simulink model "s_lqr_solar_tracking"  (R2017a)
settings: Solver=VariableStepAuto  StartTime=0.0  StopTime=10  RelTol=1e-3
values from neighbouring files (symbols this model uses):
  A = [(-R/L) (-k2/L) 0; (k1/J) 0 0; 0 1 0]    [lqr_solar_tracking.m]
  B = [(1/L); 0; 0]    [lqr_solar_tracking.m]
  C = [0 0 1]    [lqr_solar_tracking.m]
  K = lqr(A,B,Q,R)    [lqr_solar_tracking.m]
settings Model: Creator=NEGATIVE  LastModifiedBy=NEGATIVE

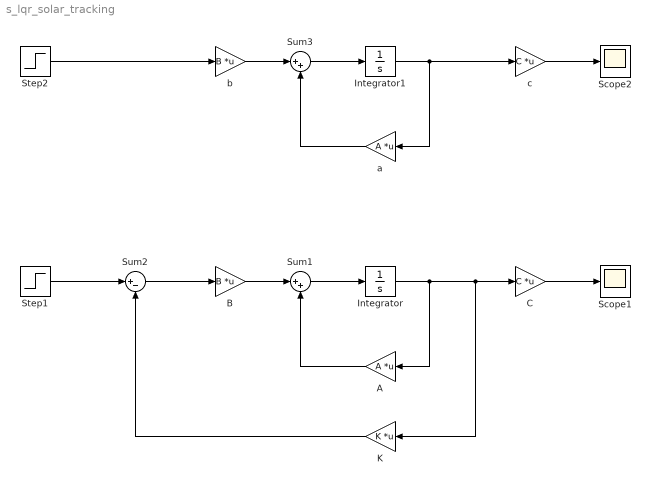
== system s_lqr_solar_tracking ==
  A : Gain  Gain=A  Multiplication=Matrix(K*u)
  B : Gain  Gain=B  Multiplication=Matrix(K*u)
  C : Gain  Gain=C  Multiplication=Matrix(K*u)
  Integrator : Integrator
  Integrator1 : Integrator
  K : Gain  Gain=K  Multiplication=Matrix(K*u)
  Scope1 : Scope
  Scope2 : Scope
  Step1 : Step  Time=0  After=24  SampleTime=0
  Step2 : Step  Time=0  After=24  SampleTime=0
  Sum1 : Sum  Inputs=|++
  Sum2 : Sum  Inputs=|+-
  Sum3 : Sum  Inputs=|++
  a : Gain  Gain=A  Multiplication=Matrix(K*u)
  b : Gain  Gain=B  Multiplication=Matrix(K*u)
  c : Gain  Gain=C  Multiplication=Matrix(K*u)
  wires:
  Sum1/1 -> Integrator/1
  B/1 -> Sum1/1
  A/1 -> Sum1/2
  Integrator/1 -> A/1, K/1, C/1
  Step1/1 -> Sum2/1
  Sum2/1 -> B/1
  K/1 -> Sum2/2
  a/1 -> Sum3/2
  b/1 -> Sum3/1
  Integrator1/1 -> a/1, c/1
  Step2/1 -> b/1
  c/1 -> Scope2/1
  Sum3/1 -> Integrator1/1
  C/1 -> Scope1/1
